simulink model "synchronusMotor"  (R2021a)
settings: Solver=ode23tb  StartTime=0.0  StopTime=120  MaxStep=500e-6  RelTol=1e-4  EnableMultiTasking=on
libraries: spsThreePhaseProgrammableVoltageSourceLib x1, spsThreePhaseSeriesRLCLoadLib x1, spsBistableLib x1, simulink x1, spsCurrentMeasurementLib x1, spsDCMachineLib x1, spsDCVoltageSourceLib x1, spsGroundLib x1, spsSeriesRLCBranchLib x1, spsSynchronousMachinepuFundamentalLib x1, spsThreePhaseVIMeasurementLib x1, spsThreePhaseBreakerLib x1
settings Model: ExtModeAutoUpdateStatusClock=off  Creator=The MathWorks, Inc.  LastModifiedBy=Abdullah123
settings SolverCC: ZeroCrossAlgorithm=Adaptive  AlgebraicLoopSolver=TrustRegion
settings DataIOCC: LimitDataPoints=on  SaveFormat=Array  ReturnWorkspaceOutputs=off
settings OptimizationCC: ExpressionDepthLimit=2147483647  InitFltsAndDblsToZero=on  EfficientMapNaN2IntZero=off  LifeSpan=inf
settings DebuggingCC: UnderspecifiedInitializationDetection=Classic  MergeDetectMultiDrivingBlocksExec=none  CheckExecutionContextPreStartOutputMsg=on  SignalResolutionControl=TryResolveAllWithWarning  SolverPrmCheckMsg=warning  MultiTaskDSMMsg=warning  MultiTaskCondExecSysMsg=none  SigSpecEnsureSampleTimeMsg=none  FcnCallInpInsideContextMsg=warning  StateNameClashWarn=warning  SFUnexpectedBacktrackingDiag=warning  SFNoUnconditionalDefaultTransitionDiag=warning  SFExecutionAtInitializationDiag=none  SFMachineParentedDataDiag=warning  ArithmeticOperatorsInVariantConditions=warning
settings HardwareCC: ProdBitPerPointer=32  ProdBitPerSizeT=32  ProdBitPerPtrDiffT=32  ProdLargestAtomicFloat=None  ProdIntDivRoundTo=Undefined  ProdEndianess=Unspecified  ProdWordSize=32  ProdHWDeviceType=32-bit Generic
settings ModelReferenceCC: PropagateSignalLabelsOutOfModel=off
settings SFSimCC: SimUseLocalCustomCode=off  CustomCodeUndefinedFunction=UseInterfaceOnly
settings RTWCC: RTWUseLocalCustomCode=off
settings CodeAppCC: StateflowObjectComments=on
settings GRTTargetCC: TargetFcnLib=ansi_tfl_tmw.mat  TargetLangStandard=C89/C90 (ANSI)  CombineOutputUpdateFcns=off  GRTInterface=on
settings ConfigComp: CovMetricSettings=dw  CovSaveCumulativeToWorkspaceVar=on  CovSaveSingleToWorkspaceVar=on  CovExternalEMLEnable=off  CovSFcnEnable=off
settings SimscapeCC: SimscapeNormalizeSystem=off

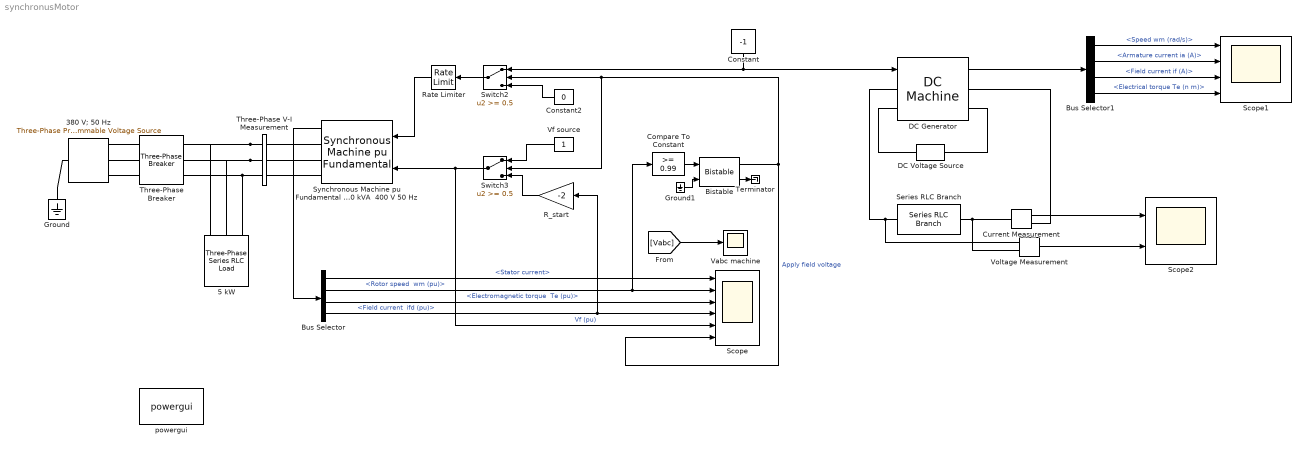
== system synchronusMotor ==
  380 V; 50 Hz : spsThreePhaseProgrammableVoltageSourceLib/Three-Phase Programmable Voltage Source  PositiveSequence="[380  0 50]"  VariationEntity=None  VariationType=Step  VariationTypeAlt=Step  VariationStep=0.5  VariationRate=10  VariationMagnitude=0.3  VariationFrequency=2  VariationTiming=[1 2]  VariationPhaseA=off  Amplitudes=[1 0.8 1.2 1.0]  TimeValues=[0 0.1 0.15 0.2]  HarmonicGeneration=off  HarmonicA=[3 0.2 -25 0]  HarmonicB=[2 0.15 35 2]  Timing="[0.05  3]"  BusType=swing  Pref=0  Qref=0  Qmin=-inf  Qmax=inf
  5 kW : spsThreePhaseSeriesRLCLoadLib/Three-Phase Series RLC Load  LConnTagsString=A|B|C  Configuration=Y (grounded)  NominalVoltage=400  Vabc=[1e3 1e3 1e3]  Vabcp=[1e3 1e3 1e3]  NominalFrequency=60  UnbalancedPower=off  ActivePower=5e3  InductivePower=0  CapacitivePower=0  Pabc=[10e3 9e3 11e3]  QLabc=[100 90 110]  QCabc=[100 90 110]  Pabcp=[10e3 9e3 11e3]  QLabcp=[100 90 110]  QCabcp=[100 90 110]  Measurements=None  LoadType=constant Z
  Bistable : spsBistableLib/Bistable  Qpriority=Set  ic=0  Ts=0
      settings: SourceProductBaseCode=PS
  Bus Selector : BusSelector  OutputSignals="Stator current,Mechanical.Rotor speed  wm (pu),Mechanical.Electromagnetic torque  Te (pu),dq0 components.Field current  ifd (pu)"
  Bus Selector1 : BusSelector  OutputSignals=Speed wm (rad/s),Armature current ia (A),Field current if (A),Electrical torque Te (n m)
  Compare To Constant : simulink/Logic and Bit Operations/Compare To Constant  relop=>=  const=0.99  OutDataTypeStr=uint8  ZeroCross=off
  Constant : Constant  Value=-1
  Constant2 : Constant  Value=0
  Current Measurement : spsCurrentMeasurementLib/Current Measurement  PhasorSimulation=off  OutputType=Complex  PSBequivalent=0
  DC Generator : spsDCMachineLib/DC Machine  PresetModel=No  MechanicalLoad=Torque TL  FieldType=Wound  ShowDetailedParameters=on  MeasurementBus=off  RLa=[2.581 0.028]  RLf=[281.3 156]  Laf=0.9483  MachineConstant=Torque constant (N.m/A)  Ke=1.8  Kt=1.8  J=0.02215  Bm=0.002953  Tf=0.5161  w0=1  Ifinit=0.355492356914326  TsPowergui=0  TsBlock=-1
  DC Voltage Source : spsDCVoltageSourceLib/DC Voltage Source  Amplitude=100  Measurements=None
  Ground : spsGroundLib/Ground  LConnTagsString=a
  Ground1 : Ground
  R_start : Gain  Gain=-2
  Rate Limiter : RateLimiter  RisingSlewLimit=3  FallingSlewLimit=-3  SampleTimeMode=inherited
  Scope : Scope  NumInputPorts=6
  Scope1 : Scope  NumInputPorts=4
  Scope2 : Scope  NumInputPorts=2
  Series RLC Branch : spsSeriesRLCBranchLib/Series RLC Branch  LConnTagsString=__new0  RConnTagsString=__new0  BranchType=R  Resistance=100  Inductance=1e-3  SetiL0=off  InitialCurrent=0  Capacitance=1e-6  Setx0=off  InitialVoltage=0  Measurements=None
  Switch2 : Switch  Threshold=0.5
  Switch3 : Switch  Threshold=0.5
  Synchronous Machine pu Fundamental 60 kVA  400 V 50 Hz : spsSynchronousMachinepuFundamentalLib/Synchronous Machine pu Fundamental  PresetModel=No  MechanicalLoad=Mechanical power Pm  ShowDetailedParameters=on  RotorType=Salient-pole  Units=per unit fundamental parameters  MeasurementBus=off  NominalParameters=[6e+004 400 50]  Stator=[0.03788 0.08 2.16 0.94]  Field=[0.02124 0.1719]  Dampers2=[0.0652, 0.5134, 0.0287, 0.2553, 7.765e-3, 0.9167 ]  Dampers1=[0.1463 0.3085 0.05754 0.05281]  Mechanical=[1.0 0.02056 2]  PolePairs=2  InitialConditions="[ -100  0  0  0  0  0  0  0  1 ]"  SetSaturation=off  Saturation=[0.6404,0.7127,0.8441,0.9214,0.9956,1.082,1.19,1.316,1.457;0.7,0.7698,0.8872,0.9466,0.9969,1.046,1.1,1.151,1.201]  LoadFlowParameters=[1,0,0,0,0]  TsPowergui=0  TsBlock=-1  IterativeModel=Trapezoidal non iterative  IterativeDiscreteModel=Trapezoidal non iterative  BusType=PV  Pref=0  Qref=0  Qmin=-inf  Qmax=inf  PLF=0  QLF=0
      settings: SourceProductBaseCode=PS
  Terminator : Terminator
  Three-Phase V-I Measurement : spsThreePhaseVIMeasurementLib/Three-Phase V-I Measurement  VoltageMeasurement=phase-to-ground  SetLabelV=on  LabelV=Vabc  Vpu=off  VpuLL=off  CurrentMeasurement=no  SetLabelI=off  LabelI=Iabc  Ipu=off  Pbase=100e6  Vbase=500e3  OutputType=Complex  PhasorSimulation=off  PSBequivalent=0
  Three-Phase Breaker : spsThreePhaseBreakerLib/Three-Phase Breaker  InitialState=open  SwitchA=on  SwitchB=on  SwitchC=on  SwitchTimes=[0.1]  External=off  BreakerResistance=0.001  SnubberResistance=1e6  SnubberCapacitance=inf  Measurements=None
  Vabc machine : Scope
  Vf source : Constant
  Voltage Measurement : spsVoltageMeasurementLib/Voltage Measurement  PhasorSimulation=off  OutputType=Complex  PSBequivalent=0
  powergui : spspowerguiLib/powergui  Priority=2  SimulationMode=Continuous  SampleTime=0  frequency=60  Iterations=50  frequencyindice=0  Pbase=100e6  ErrMax=1e-4  UnitsV=kV  UnitsW=MW  buscounter=0  FunctionMessages=off  echomessages=off  EnableUseOfTLC=off  CurrentSourceSwitches=off  DisableSnubberDevices=off  DisableRonSwitches=off  DisableVfSwitches=off  DisplayEquations=off  AutomaticDiscreteSolvers=off  SolverType=Tustin  Interpol=off  ExternalGateDelay=off  methode=off  Ts=0  x0status=blocks  SPID=on  SwTol=0  HookPort=off  NonlinearTolerance=1e-4  nMaxIteration=100  ContinueOnMaxIteration=off  RestoreLinks=warning  ResistiveCurrentMeasurement=off  Frange=[0:2:500]  Ylog=off  Xlog=on  ShowGrid=off  save=off  variable=ZData  structure=0  ZoomFFT=on  StartTime=0.0  cycles=1  DisplayStyle=1  fundamental=60  FreqAxis=off  MaxFrequency=1000  frequencyindicesteady=1  RmsSteady=1  display=off
  wires:
  Bus Selector/1 -> Scope/1  "<Stator current>"
  Bus Selector/2 -> Scope/2, Compare To Constant/1  "<Rotor speed  wm (pu)>"
  Bus Selector/3 -> Scope/3  "<Electromagnetic torque  Te (pu)>"
  Bus Selector/4 -> Scope/4, R_start/1  "<Field current  ifd (pu)>"
  Switch3/1 -> Scope/5, Synchronous Machine pu Fundamental 60 kVA  400 V 50 Hz/2  "Vf (pu)"
  Switch2/1 -> Rate Limiter/1
  Rate Limiter/1 -> Synchronous Machine pu Fundamental 60 kVA  400 V 50 Hz/1
  Synchronous Machine pu Fundamental 60 kVA  400 V 50 Hz/1 -> Bus Selector/1
  Bistable/2 -> Terminator/1
  Constant2/1 -> Switch2/3
  Vf source/1 -> Switch3/1
  R_start/1 -> Switch3/3
  Ground1/1 -> Bistable/2
  Compare To Constant/1 -> Bistable/1
  Bistable/1 -> Scope/6, Switch2/2, Switch3/2  "Apply field voltage"
  [Vabc] -> Vabc machine/1
  Constant/1 -> Switch2/1, DC Generator/1
  DC Generator/1 -> Bus Selector1/1
  Bus Selector1/1 -> Scope1/1  "<Speed wm (rad/s)>"
  Bus Selector1/2 -> Scope1/2  "<Armature current ia (A)>"
  Bus Selector1/3 -> Scope1/3  "<Field current if (A)>"
  Bus Selector1/4 -> Scope1/4  "<Electrical torque Te (n m)>"
  Current Measurement/1 -> Scope2/1
  Voltage Measurement/1 -> Scope2/2
  connections:
  380 V; 50 Hz/RConn1 -- Three-Phase Breaker/LConn1
  380 V; 50 Hz/RConn2 -- Three-Phase Breaker/LConn2
  380 V; 50 Hz/RConn3 -- Three-Phase Breaker/LConn3
  Three-Phase V-I Measurement/LConn1 -- 5 kW/LConn1 -- Three-Phase Breaker/RConn1
  Three-Phase V-I Measurement/LConn2 -- 5 kW/LConn2 -- Three-Phase Breaker/RConn2
  5 kW/LConn3 -- Three-Phase Breaker/RConn3 -- Three-Phase V-I Measurement/LConn3
  Ground/LConn1 -- 380 V; 50 Hz/LConn1
  Three-Phase V-I Measurement/RConn3 -- Synchronous Machine pu Fundamental 60 kVA  400 V 50 Hz/RConn3
  Three-Phase V-I Measurement/RConn1 -- Synchronous Machine pu Fundamental 60 kVA  400 V 50 Hz/RConn1
  Three-Phase V-I Measurement/RConn2 -- Synchronous Machine pu Fundamental 60 kVA  400 V 50 Hz/RConn2
  DC Generator/LConn2 -- DC Voltage Source/RConn1
  DC Generator/RConn2 -- DC Voltage Source/LConn1
  DC Generator/LConn1 -- Voltage Measurement/LConn1 -- Series RLC Branch/LConn1
  Current Measurement/LConn1 -- Voltage Measurement/LConn2 -- Series RLC Branch/RConn1
  Current Measurement/RConn1 -- DC Generator/RConn1
